simulink model "Reforce_Experiment_FCS"  (R2021a)
settings: Solver=FixedStepDiscrete  StartTime=0.0  StopTime=Inf  FixedStep=Ts  RelTol=1e-3
PostLoadFcn:
  | , if any(exist('dsrtsu_mdlpostloadfcn', 'file') ~= 0), dsrtsu_mdlpostloadfcn('Execute', bdroot); end,
InitFcn:
  | , if any(exist('rtifpga_mdlclblib', 'file') ~= 0), rtifpga_mdlclblib('Init', bdroot); end,
model workspace (MAT data in the model file):
  FPGA_Control_Scheme_1_Buffer_1_1_1_write : Simulink.Signal (value not decoded)
  FPGA_Control_Scheme_1_Buffer_2_1_1_write : Simulink.Signal (value not decoded)
  FPGA_Control_Scheme_1_Register_1_1_1_write : Simulink.Signal (value not decoded)
  FPGA_Control_Scheme_1_Register_2_1_1_write : Simulink.Signal (value not decoded)
values from neighbouring files (symbols this model uses):
  abc2alphabeta0 = [      2/3      -1/3       -1/3 ... (first row only)    [Reforce_Init_FCS.m]
  alphabeta02abc = [  1          0 1/sqrt(2) ... (first row only)    [Reforce_Init_FCS.m]
  torque_ref_sample_lower = -torque_ref_sample_upper    (= -6.5)    [Reforce_Init_FCS.m]
  torque_ref_sample_upper = 6.5    [Reforce_Init_FCS.m]
  Ts = 50e-6    (= 5e-05)    [Reforce_Init_FCS.m]
  uf_factor = U_nom / f_nom    (= 2.82)    [Reforce_Init_FCS.m]
undefined symbols (not defined in the file or in its folder): CC, controller, init_layer_0, init_layer_1, init_layer_2, init_layer_3, init_layer_4, init_layer_5, init_layer_6, init_layer_7, init_layer_8, init_layer_9, inverter, load, motor, PLL, sensor
libraries: simulink x16, rtiproclib x13, rti1202lib_adc_class1 x8, rti1202lib_dio_class1 x4, dspfdesign x3, rtiemclib x2, rti1202lib_dac_class1 x1, embmathops x1, rti1202lib_base x1, rtitasklib x1, dsextras x1, simulink_extras x1
(part 2 of 6)

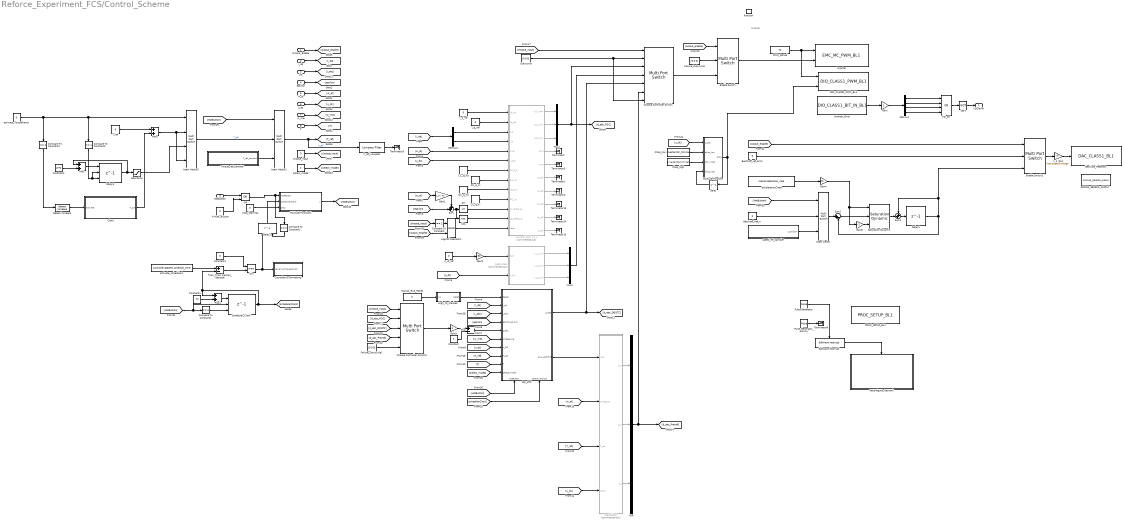
== system Reforce_Experiment_FCS/Control_Scheme ==
  note: Inverter
  Output_Enable : Inport
  i_dq : Inport  Port=2
  In3 : Inport  Port=3
  epsilon : Inport  Port=4
  w_el : Inport  Port=5
  u_dc : Inport  Port=6
  w_me : Inport  Port=7
  T : Inport  Port=8
  HotButton : Inport  Port=9
  function : TriggerPort  TriggerType=function-call  VariantControl=(inherit)
  Add : Sum
  Add1 : Sum
  Beckhoff_Ref_n : Constant  Value=0
  Beckhoff_Referenz : rti1202lib_dac_class1/DAC_CLASS1_BL1  DSProperties=struct('RTI',struct('Version',uint32(2),'BlockType',struct('isSLSource',uint8(0),'isSLSink',uint8(1),'isHWSource',uint8(0),'isHWSink',uint8(1),'isSetup',uint8(0),'isInline',uint8(1),'isNonInline',uint8(0),'isInterrupt',uint8(0),'isChannelwise',uint8(1)),'IOBoardType',{{'DS120X','STD','DACC1'}},'UnitType','DAC','Identifier','DAC','DialogType','ML','BlockSet','NONE','SlaveProcessor','NONE'))  RTIBlockInterface=struct('InputPortsActive',1,'InputPortsWidth',int32(1),'InputPortsDataType',{{'SS_DOUBLE'}},'InputPortsName',{{['DAC 8']}},'DialogFcn','rti120xstddacc1dacgui','InitLevel',3,'IconTransparency','on','BlockDisplay',{{['DAC CL1\nChannel: 8'],'center'}},'BlockName',struct('Token',{{'DAC_CLASS1_BL1'}}))  RTIBlockParameters=struct('ChannelNo',{{8,'OFF',[]}},'ChannelNumOf',{{1,'OFF',[]}},'InitialValue1',{{'0','OFF',[-10 10]}},'InitialValue2',{{'0','OFF',[-10 10]}},'InitialValue3',{{'0','OFF',[-10 10]}},'InitialValue4',{{'0','OFF',[-10 10]}},'InitialValue5',{{'0','OFF',[-10 10]}},'InitialValue6',{{'0','OFF',[-10 10]}},'InitialValue7',{{'0','OFF',[-10 10]}},'InitialValue8',{{'0','OFF',[-10 10]}},'InitialValue9',{{'0','OFF',[-10 10]}},'InitialValue10',{{'0','OFF',[-10 10]}},'InitialValue11',{{'0','OFF',[-10 10]}},'InitialValue12',{{'0','OFF',[-10 10]}},'InitialValue13',{{'0','OFF',[-10 10]}},'InitialValue14',{{'0','OFF',[-10 10]}},'InitialValue15',{{'0','OFF',[-10 10]}},'InitialValue16',{{'0','OFF',[-10 10]}},'OutputMode',{{[2 1 1 1 1 1 1 1 1 1 1 1 1 1 1 1],'OFF',[1 2]}},'TermValue1',{{'0','OFF',[-10 10]}},'TermValue2',{{'0','OFF',[-10 10]}},'TermValue3',{{'0','OFF',[-10 10]}},'TermValue4',{{'0','OFF',[-10 10]}},'TermValue5',{{'0','OFF',[-10 10]}},'TermValue6',{{'0','OFF',[-10 10]}},'TermValue7',{{'0','OFF',[-10 10]}},'TermValue8',{{'0','OFF',[-10 10]}},'TermValue9',{{'0','OFF',[-10 10]}},'TermValue10',{{'0','OFF',[-10 10]}},'TermValue11',{{'0','OFF',[-10 10]}},'TermValue12',{{'0','OFF',[-10 10]}},'TermValue13',{{'0','OFF',[-10 10]}},'TermValue14',{{'0','OFF',[-10 10]}},'TermValue15',{{'0','OFF',[-10 10]}},'TermValue16',{{'0','OFF',[-10 10]}},'EnableTermMode',{{1,'OFF',[0 1]}},'TLCFileName',{{'rti120xdac_c1_dac','OFF',[]}},'InitialValueBuildCheck1',{{0,'OFF',[]}},'InitialValueBuildCheck2',{{0,'OFF',[]}},'InitialValueBuildCheck3',{{0,'OFF',[]}},'InitialValueBuildCheck4',{{0,'OFF',[]}},'InitialValueBuildCheck5',{{0,'OFF',[]}},'InitialValueBuildCheck6',{{0,'OFF',[]}},'InitialValueBuildCheck7',{{0,'OFF',[]}},'InitialValueBuildCheck8',{{1,'OFF',[]}},'InitialValueBuildCheck9',{{0,'OFF',[]}},'InitialValueBuildCheck10',{{0,'OFF',[]}},'InitialValueBuildCheck11',{{0,'OFF',[]}},'InitialValueBuildCheck12',{{0,'OFF',[]}},'InitialValueBuildCheck13',{{0,'OFF',[]}},'InitialValueBuildCheck14',{{0,'OFF',[]}},'InitialValueBuildCheck15',{{0,'OFF',[]}},'InitialValueBuildCheck16',{{0,'OFF',[]}},'TermValueBuildCheck1',{{0,'OFF',[]}},'TermValueBuildCheck2',{{0,'OFF',[]}},'TermValueBuildCheck3',{{0,'OFF',[]}},'TermValueBuildCheck4',{{0,'OFF',[]}},'TermValueBuildCheck5',{{0,'OFF',[]}},'TermValueBuildCheck6',{{0,'OFF',[]}},'TermValueBuildCheck7',{{0,'OFF',[]}},'TermValueBuildCheck8',{{0,'OFF',[]}},'TermValueBuildCheck9',{{0,'OFF',[]}},'TermValueBuildCheck10',{{0,'OFF',[]}},'TermValueBuildCheck11',{{0,'OFF',[]}},'TermValueBuildCheck12',{{0,'OFF',[]}},'TermValueBuildCheck13',{{0,'OFF',[]}},'TermValueBuildCheck14',{{0,'OFF',[]}},'TermValueBuildCheck15',{{0,'OFF',[]}},'TermValueBuildCheck16',{{0,'OFF',[]}})  RTISFcnParameters=struct('ChannelNo','int16','ChannelNumOf','int16','InitialValue1','double','InitialValue2','double','InitialValue3','double','InitialValue4','double','InitialValue5','double','InitialValue6','double','InitialValue7','double','InitialValue8','double','InitialValue9','double','InitialValue10','double','InitialValue11','double','InitialValue12','double','InitialValue13','double','InitialValue14','double','InitialValue15','double','InitialValue16','double','OutputMode','int16','TermValue1','double','TermValue2','double','TermValue3','double','TermValue4','double','TermValue5','double','TermValue6','double','TermValue7','double','TermValue8','double','TermValue9','double','TermValue10','double','TermValue11','double','TermValue12','double','TermValue13','double','TermValue14','double','TermValue15','double','TermValue16','double','EnableTermMode','int16','TLCFileName','char')  RTIBlockParaDefault=struct('ChannelNo',1,'ChannelNumOf',1,'InitialValue1',0,'InitialValue2',0,'InitialValue3',0,'InitialValue4',0,'InitialValue5',0,'InitialValue6',0,'InitialValue7',0,'InitialValue8',0,'InitialValue9',0,'InitialValue10',0,'InitialValue11',0,'InitialValue12',0,'InitialValue13',0,'InitialValue14',0,'InitialValue15',0,'InitialValue16',0,'OutputMode',ones(1,16),'TermValue1',0,'TermValue2',0,'TermValue3',0,'TermValue4',0,'TermValue5',0,'TermValue6',0,'TermValue7',0,'TermValue8',0,'TermValue9',0,'TermValue10',0,'TermValue11',0,'TermValue12',0,'TermValue13',0,'TermValue14',0,'TermValue15',0,'TermValue16',0,'EnableTermMode',0,'TLCFileName','rti120xdac_c1_dac','InitialValueBuildCheck1',0,'InitialValueBuildCheck2',0,'InitialValueBuildCheck3',0,'InitialValueBuildCheck4',0,'InitialValueBuildCheck5',0,'InitialValueBuildCheck6',0,'InitialValueBuildCheck7',0,'InitialValueBuildCheck8',0,'InitialValueBuildCheck9',0,'InitialValueBuildCheck10',0,'InitialValueBuildCheck11',0,'InitialValueBuildCheck12',0,'InitialValueBuildCheck13',0,'InitialValueBuildCheck14',0,'InitialValueBuildCheck15',0,'InitialValueBuildCheck16',0,'TermValueBuildCheck1',0,'TermValueBuildCheck2',0,'TermValueBuildCheck3',0,'TermValueBuildCheck4',0,'TermValueBuildCheck5',0,'TermValueBuildCheck6',0,'TermValueBuildCheck7',0,'TermValueBuildCheck8',0,'TermValueBuildCheck9',0,'TermValueBuildCheck10',0,'TermValueBuildCheck11',0,'TermValueBuildCheck12',0,'TermValueBuildCheck13',0,'TermValueBuildCheck14',0,'TermValueBuildCheck15',0,'TermValueBuildCheck16',0)
  Beckhoff_ref_error : Constant  Value=0
  CC_d_Ki : Constant  Value=CC.d.Ki
  CC_d_Kp : Constant  Value=CC.d.Kp
  CC_q_Ki : Constant  Value=CC.q.Ki
  CC_q_Kp : Constant  Value=CC.q.Kp
  Chart : Stateflow chart  TreatAsAtomicUnit=on
  Choose Controller Switch : MultiPortSwitch  DataPortOrder=Zero-based contiguous  Inputs=5  DataPortForDefault=Additional data port  zeroidx=on
  Choose Controller Switch1 : MultiPortSwitch  DataPortOrder=Specify indices  Inputs=5  DataPortIndices={1,3,4}  DataPortForDefault=Additional data port  DiagnosticForDefault=None
  Chop_high : Constant  Value=inverter.DC_link.high
  Chop_low : Constant  Value=inverter.DC_link.low
  Compare To Constant : simulink/Logic and Bit Operations/Compare To Constant  relop===  const=1  OutDataTypeStr=boolean
  Compare To Constant1 : simulink/Logic and Bit Operations/Compare To Constant  relop===  const=0  OutDataTypeStr=boolean
  Compare To Constant2 : simulink/Logic and Bit Operations/Compare To Constant  relop===  const=0  OutDataTypeStr=boolean
  Compare To Constant3 : simulink/Logic and Bit Operations/Compare To Constant  relop===  const=1  OutDataTypeStr=boolean
  Compare To Constant4 : simulink/Logic and Bit Operations/Compare To Constant  relop===  const=2  OutDataTypeStr=boolean
  Constant : Constant
  Constant1 : Constant  Value=Ts
  Constant2 : Constant  Value=4*Ts
  Constant4 : Constant  Value=0
  Cos : Trigonometry  Operator=cos  NumberOfDataPoints=64
  Countdown_Formatting : Subsystem
  DIO_CLASS1_PWM_BL1 : rti1202lib_dio_class1/DIO_CLASS1_PWM_BL1  DSProperties=struct('RTI',struct('Version',uint32(1),'BlockType',struct('isSLSource',uint8(0),'isSLSink',uint8(1),'isHWSource',uint8(0),'isHWSink',uint8(1),'isSetup',uint8(0),'isInline',uint8(1),'isNonInline',uint8(0),'isInterrupt',uint8(0),'isChannelwise',uint8(1)),'IOBoardType',{{'DS120X','STD','DIOC1'}},'UnitType','PWM','Identifier','PWM','DialogType','ML','BlockSet','NONE','SlaveProcessor','NONE'))  RTIBlockInterface=struct('InputPortsWidth',int32([1 1]),'InputPortsActive',[1 1],'InputPortsName',{{'Period',['Duty Cycle']}},'BlockDisplay',{{['DIO CL1 PWM\nPort: 1\nChannel: 7'],'center'}},'IconTransparency','on','InitLevel',3,'DialogFcn','rti120xstddioc1pwmgui','BlockName',struct('Token',{{'DIO_CLASS1_PWM_BL1'}}))  RTIBlockParameters=struct('PortNo',{{1,'OFF',[]}},'ChannelNo',{{7,'OFF',[]}},'HighLevel',{{2,'OFF',[1 3]}},'UpdateMode',{{1,'OFF',[1 2]}},'InvertingMode',{{1,'OFF',[1 2]}},'DutyCycleInit',{{'0.0','OFF',[0 1]}},'DutyCycleTerm',{{'0','OFF',[0 1]}},'PeriodInit',{{'Ts','OFF',[1e-7 1.34]}},'PeriodTerm',{{'Ts','OFF',[1e-7 1.34]}},'TerminationMode',{{1,'OFF',[0 1]}},'OutputTermValidate',{{1,'OFF',[0 1]}},'OutputTermBuildCheck',{{true,'OFF',[]}},'EnableEvent',{{0,'OFF',[0 1]}},'EventMode',{{1,'OFF',[1 3]}},'EventOnFalling',{{1,'OFF',[0 1]}},'EventOnRising',{{0,'OFF',[0 1]}},'EventDelay',{{'0','OFF',[0 1.34]}},'EventRate',{{'1','OFF',[1 256]}},'EventBuildCheck',{{false,'OFF',[]}},'TriggerLine',{{1,'OFF',[1 16]}},'TLCFileName',{{'rti120xdio_c1_pwm','OFF',[]}})  RTISFcnParameters=struct('PortNo','int16','ChannelNo','int16','HighLevel','int16','UpdateMode','int16','InvertingMode','int16','DutyCycleInit','double','DutyCycleTerm','double','PeriodInit','double','PeriodTerm','double','TerminationMode','int16','OutputTermValidate','int16','EnableEvent','int16','EventMode','int16','EventOnFalling','int16','EventOnRising','int16','EventDelay','double','EventRate','int16','TriggerLine','int16','TLCFileName','char')  RTIBlockParaDefault=struct('PortNo',1,'ChannelNo',1,'HighLevel',1,'UpdateMode',1,'InvertingMode',1,'DutyCycleInit',2^-1,'DutyCycleTerm',2^-1,'PeriodInit',5e-5,'PeriodTerm',5e-5,'TerminationMode',0,'OutputTermValidate',0,'OutputTermBuildCheck',0,'EnableEvent',0,'EventMode',1,'EventOnFalling',1,'EventOnRising',0,'EventDelay',0,'EventRate',1,'EventBuildCheck',0,'TriggerLine',1,'TLCFileName','rti120xdio_c1_pwm')
  DQ_DTC : Subsystem
      settings: PortSchema="{\"entries\":[{\"content\":{\"sides\":[{\"content\":{\"connectorIds\":[\"In1\",\"In2\",\"In3\",\"In4\",\"In5\",\"In6\",\"In7\",\"In8\",\"In9\",\"In10\"]},\"type\":\"ConnectorPlacement.EquallySpacedRectSide\",\"uuid\":\"02ff152a-d5e9-48ae-8ae9-04f46c283eee\"},{\"content\":{\"connectorIds\":[\"Out1\",\"Out2\"],\"side\":\"RIGHT\"},\"type\":\"ConnectorPlacement.EquallySpacedRectSide\",\"uuid\":\"642da27a-b041-4256-941e-23b0305d4ed5\"},{\"content\":{\"connectorIds\":[],\"side\":\"TOP\"},\"type\":\"ConnectorPlacement.EquallySpacedRectSide\",\"uuid\":\"a1b72579-caca-49f6-8122-3333a1b1b672\"},{\"content\":{\"connectorIds\":[\"In11\",\"In12\"],\"side\":\"BOTTOM\"},\"type\":\"ConnectorPlacement.EquallySpacedRectSide\",\"uuid\":\"d4b983f3-21ae-48af-86f0-0aec95f79f6c\"}]},\"type\":\"ConnectorPlacement.EquallySpacedConnector\",\"uuid\":\"9d77db4d-e82d-471c-b407-1ac7a7d31965\"}],\"packageUris\":[\"http://schema.mathworks.com/mf0/Connector/R2020b\"],\"version\":\"1.0\"}"
  DS1202_SENSOR_SUPPLY : rti1202lib_base/DS1202_SENSOR_SUPPLY  DSProperties=struct('RTI',struct('Version',uint32(1),'BlockType',struct('isSLSource',uint8(0),'isSLSink',uint8(0),'isHWSource',uint8(0),'isHWSink',uint8(1),'isSetup',uint8(0),'isInline',uint8(1),'isNonInline',uint8(0),'isInterrupt',uint8(0),'isChannelwise',uint8(0)),'IOBoardType',{{'DS120X','BASE'}},'UnitType','SENSORSUPPLY','Identifier','SENSORSUPPLY','DialogType','ML','BlockSet','NONE','SlaveProcessor','NONE'))  RTIBlockInterface=struct('OutputPortsActive',0,'OutputPortsWidth',int32(0),'DialogFcn','rti120xbasesensorsupplygui','InitLevel',3,'IconTransparency','off','BlockDisplay',{{['DS1202\nSensor Supply'],'center'}},'BlockName',struct('Token',{{'DS1202_SENSOR_SUPPLY'}}))  RTIBlockParameters=struct('Voltage',{{2,'OFF',[2 20]}},'TLCFileName',{{'rti120xbase_sensor_supply','OFF',[]}})  RTISFcnParameters=struct('Voltage','double','TLCFileName','char')  RTIBlockParaDefault=struct('Voltage',2,'TLCFileName','rti120xbase_sensor_supply')
  Delay : Delay  DelayLength=1
  Delay1 : Delay  DelayLength=1  InitialCondition=0
  Delay2 : Delay  DelayLength=1  InitialCondition=controller.DQDTC.schedule_time  ExternalReset=Either
      settings: InputPortMap=u0,r5
  Delay3 : Delay  DelayLength=1  InitialCondition=-5  ExternalReset=Either  ShowEnablePort=on
      settings: InputPortMap=u0,e6,r5
  Demux1 : Demux
  Demux2 : Demux  Outputs=2
  Detect Increase : simulink/Logic and Bit Operations/Detect Increase  vinit=0.0  OutDataTypeStr=boolean
  Dutycycle : Constant  Value=[0 0 0]
  Enable Switch : MultiPortSwitch  DataPortOrder=Zero-based contiguous  Inputs=2  zeroidx=on
  Enable Switch1 : MultiPortSwitch  DataPortOrder=Zero-based contiguous  Inputs=2  zeroidx=on
  Failure_Dutycycle : Constant  Value=[0 0 0]
  Failure_Dutycycle1 : Constant  Value=[0 0 0]
  Gain : Gain
  Gain1 : Gain  Gain=1.5 * Ts
  Gain2 : Gain  Gain=60
  Gain3 : Gain  Gain=2
  Gain4 : Gain  Gain=Ts
  Gain5 : Gain  Gain=-1
  High_To_Flanke3 : Subsystem
  Index Vector : MultiPortSwitch  DataPortOrder=Zero-based contiguous  Inputs=2  zeroidx=on
  Index Vector1 : MultiPortSwitch  DataPortOrder=Zero-based contiguous  Inputs=2  zeroidx=on
  Index Vector2 : MultiPortSwitch  DataPortOrder=Zero-based contiguous  zeroidx=on
  Inverter : rtiemclib/EMC_MC_PWM_BL1  DSProperties=struct('RTI',struct('Version',uint32(2),'BlockType',struct('isSLSource',uint8(0),'isSLSink',uint8(1),'isHWSource',uint8(0),'isHWSink',uint8(1),'isSetup',uint8(0),'isInline',uint8(1),'isNonInline',uint8(0),'isInterrupt',uint8(0),'isChannelwise',uint8(1)),'IOBoardType','DSEMC','UnitType','MCPWM','Identifier','MCPWM','DialogType','ML','BlockSet','RTIEMC','SlaveProcessor','NONE'))  RTIBlockInterface=struct('InputPortsWidth',int32([1 3 1]),'InputPortsActive',[1 1 0],'InputPortsName',{{'Period',['Duty Cycle'],['Output Enable']}},'BlockDisplay',{{['EMC Multi Channel PWM\nPort: 1\nChannel: 1\nNumber of channels: 3'],'center'}},'IconTransparency','on','InitLevel',3,'DialogFcn','rtiemcmcpwmgui','BlockName',struct('Token',{{'EMC_MC_PWM_BL1'}}),'InputPortsDataType',{{'SS_DOUBLE','SS_DOUBLE','SS_BOOLEAN'}})  RTIBlockParameters=struct('PortNo',{{1,'OFF',[1 3]}},'ChannelNo',{{1,'OFF',[1 16]}},'InvChannelMode',{{2,'OFF',[1 2]}},'NumOfChannels',{{3,'OFF',[1 8]}},'HighLevel',{{2,'OFF',[1 3]}},'AlignmentMode',{{2,'OFF',[1 2]}},'UpdateModeCA',{{1,'OFF',[1 3]}},'UpdateModeEA',{{2,'OFF',[1 2]}},'DeadTime',{{'5e-6','OFF',[0 0.000655]}},'InitPeriod',{{'50e-6','OFF',[1e-7 1.34]}},'InitDutyCycle1',{{'0','OFF',[0 1]}},'InitDutyCycle2',{{'0','OFF',[0 1]}},'InitDutyCycle3',{{'0','OFF',[0 1]}},'InitDutyCycle4',{{'0.5','OFF',[0 1]}},'InitDutyCycle5',{{'0.5','OFF',[0 1]}},'InitDutyCycle6',{{'0.5','OFF',[0 1]}},'InitDutyCycle7',{{'0.5','OFF',[0 1]}},'InitDutyCycle8',{{'0.5','OFF',[0 1]}},'InitDutyCycle9',{{'0.5','OFF',[0 1]}},'InitDutyCycle10',{{'0.5','OFF',[0 1]}},'InitDutyCycle11',{{'0.5','OFF',[0 1]}},'InitDutyCycle12',{{'0.5','OFF',[0 1]}},'InitDutyCycle13',{{'0.5','OFF',[0 1]}},'InitDutyCycle14',{{'0.5','OFF',[0 1]}},'InitDutyCycle15',{{'0.5','OFF',[0 1]}},'InitDutyCycle16',{{'0.5','OFF',[0 1]}},'TerminationMode',{{1,'OFF',[0 1]}},'OutputTermValidate',{{1,'OFF',[0 1]}},'TermPeriod',{{'50e-06','OFF',[1e-7 1.34]}},'TermDutyCycle1',{{'0','OFF',[0 1]}},'TermDutyCycle2',{{'0','OFF',[0 1]}},'TermDutyCycle3',{{'0','OFF',[0 1]}},'TermDutyCycle4',{{'0.5','OFF',[0 1]}},'TermDutyCycle5',{{'0.5','OFF',[0 1]}},'TermDutyCycle6',{{'0.5','OFF',[0 1]}},'TermDutyCycle7',{{'0.5','OFF',[0 1]}},'TermDutyCycle8',{{'0.5','OFF',[0 1]}},'TermDutyCycle9',{{'0.5','OFF',[0 1]}},'TermDutyCycle10',{{'0.5','OFF',[0 1]}},'TermDutyCycle11',{{'0.5','OFF',[0 1]}},'TermDutyCycle12',{{'0.5','OFF',[0 1]}},'TermDutyCycle13',{{'0.5','OFF',[0 1]}},'TermDutyCycle14',{{'0.5','OFF',[0 1]}},'TermDutyCycle15',{{'0.5','OFF',[0 1]}},'TermDutyCycle16',{{'0.5','OFF',[0 1]}},'EnableEvent',{{0,'OFF',[0 1]}},'EventMode',{{3,'OFF',[1 3]}},'EventOnStart',{{1,'OFF',[0 1]}},'EventOnCenter',{{0,'OFF',[0 1]}},'EventDelay',{{'25e-6','OFF',[0 1.34]}},'EventRate',{{'1','OFF',[1 256]}},'TriggerLine',{{1,'OFF',[1 16]}},'TLCFileName',{{'rtiemcmcpwm','OFF',[]}},'ValidateDeadTimeBuildCheck',{{false,'OFF',[]}},'InitDutyCycleBuildCheck1',{{1,'OFF',[]}},'InitDutyCycleBuildCheck2',{{1,'OFF',[]}},'InitDutyCycleBuildCheck3',{{1,'OFF',[]}},'InitDutyCycleBuildCheck4',{{0,'OFF',[]}},'InitDutyCycleBuildCheck5',{{0,'OFF',[]}},'InitDutyCycleBuildCheck6',{{0,'OFF',[]}},'InitDutyCycleBuildCheck7',{{0,'OFF',[]}},'InitDutyCycleBuildCheck8',{{0,'OFF',[]}},'InitDutyCycleBuildCheck9',{{0,'OFF',[]}},'InitDutyCycleBuildCheck10',{{0,'OFF',[]}},'InitDutyCycleBuildCheck11',{{0,'OFF',[]}},'InitDutyCycleBuildCheck12',{{0,'OFF',[]}},'InitDutyCycleBuildCheck13',{{0,'OFF',[]}},'InitDutyCycleBuildCheck14',{{0,'OFF',[]}},'InitDutyCycleBuildCheck15',{{0,'OFF',[]}},'InitDutyCycleBuildCheck16',{{0,'OFF',[]}},'ValidateTermBuildCheck',{{true,'OFF',[]}},'TermDutyCycleBuildCheck1',{{1,'OFF',[]}},'TermDutyCycleBuildCheck2',{{1,'OFF',[]}},'TermDutyCycleBuildCheck3',{{1,'OFF',[]}},'TermDutyCycleBuildCheck4',{{0,'OFF',[]}},'TermDutyCycleBuildCheck5',{{0,'OFF',[]}},'TermDutyCycleBuildCheck6',{{0,'OFF',[]}},'TermDutyCycleBuildCheck7',{{0,'OFF',[]}},'TermDutyCycleBuildCheck8',{{0,'OFF',[]}},'TermDutyCycleBuildCheck9',{{0,'OFF',[]}},'TermDutyCycleBuildCheck10',{{0,'OFF',[]}},'TermDutyCycleBuildCheck11',{{0,'OFF',[]}},'TermDutyCycleBuildCheck12',{{0,'OFF',[]}},'TermDutyCycleBuildCheck13',{{0,'OFF',[]}},'TermDutyCycleBuildCheck14',{{0,'OFF',[]}},'TermDutyCycleBuildCheck15',{{0,'OFF',[]}},'TermDutyCycleBuildCheck16',{{0,'OFF',[]}},'ValidateEventBuildCheck',{{false,'OFF',[]}},'ActivateOutputEnablePort',{{0,'OFF',[0 1]}},'InitOutputEnable',{{2,'OFF',[1 2]}})  RTISFcnParameters=struct('PortNo','int32','ChannelNo','int32','InvChannelMode','int32','NumOfChannels','int32','HighLevel','int32','AlignmentMode','int32','UpdateModeCA','int32','UpdateModeEA','int32','DeadTime','double','InitPeriod','double','InitDutyCycle1','double','InitDutyCycle2','double','InitDutyCycle3','double','InitDutyCycle4','double','InitDutyCycle5','double','InitDutyCycle6','double','InitDutyCycle7','double','InitDutyCycle8','double','InitDutyCycle9','double','InitDutyCycle10','double','InitDutyCycle11','double','InitDutyCycle12','double','InitDutyCycle13','double','InitDutyCycle14','double','InitDutyCycle15','double','InitDutyCycle16','double','TerminationMode','uint32','OutputTermValidate','int32','TermPeriod','double','TermDutyCycle1','double','TermDutyCycle2','double','TermDutyCycle3','double','TermDutyCycle4','double','TermDutyCycle5','double','TermDutyCycle6','double','TermDutyCycle7','double','TermDutyCycle8','double','TermDutyCycle9','double','TermDutyCycle10','double','TermDutyCycle11','double','TermDutyCycle12','double','TermDutyCycle13','double','TermDutyCycle14','double','TermDutyCycle15','double','TermDutyCycle16','double','EnableEvent','int32','EventMode','int32','EventOnStart','int32','EventOnCenter','int32','EventDelay','double','EventRate','int32','TriggerLine','int32','TLCFileName','char','ActivateOutputEnablePort','int32','InitOutputEnable','int32')  RTIBlockParaDefault=struct('PortNo',1,'ChannelNo',1,'InvChannelMode',1,'NumOfChannels',1,'HighLevel',1,'AlignmentMode',1,'UpdateModeCA',1,'UpdateModeEA',1,'DeadTime',0,'InitPeriod',5e-5,'InitDutyCycle1',2^-1,'InitDutyCycle2',2^-1,'InitDutyCycle3',2^-1,'InitDutyCycle4',2^-1,'InitDutyCycle5',2^-1,'InitDutyCycle6',2^-1,'InitDutyCycle7',2^-1,'InitDutyCycle8',2^-1,'InitDutyCycle9',2^-1,'InitDutyCycle10',2^-1,'InitDutyCycle11',2^-1,'InitDutyCycle12',2^-1,'InitDutyCycle13',2^-1,'InitDutyCycle14',2^-1,'InitDutyCycle15',2^-1,'InitDutyCycle16',2^-1,'TerminationMode',0,'OutputTermValidate',0,'TermPeriod',5e-5,'TermDutyCycle1',2^-1,'TermDutyCycle2',2^-1,'TermDutyCycle3',2^-1,'TermDutyCycle4',2^-1,'TermDutyCycle5',2^-1,'TermDutyCycle6',2^-1,'TermDutyCycle7',2^-1,'TermDutyCycle8',2^-1,'TermDutyCycle9',2^-1,'TermDutyCycle10',2^-1,'TermDutyCycle11',2^-1,'TermDutyCycle12',2^-1,'TermDutyCycle13',2^-1,'TermDutyCycle14',2^-1,'TermDutyCycle15',2^-1,'TermDutyCycle16',2^-1,'EnableEvent',0,'EventMode',1,'EventOnStart',1,'EventOnCenter',0,'EventDelay',0,'EventRate',1,'TriggerLine',1,'TLCFileName','rtiemcmcpwm','ValidateDeadTimeBuildCheck',0,'InitDutyCycleBuildCheck1',0,'InitDutyCycleBuildCheck2',0,'InitDutyCycleBuildCheck3',0,'InitDutyCycleBuildCheck4',0,'InitDutyCycleBuildCheck5',0,'InitDutyCycleBuildCheck6',0,'InitDutyCycleBuildCheck7',0,'InitDutyCycleBuildCheck8',0,'InitDutyCycleBuildCheck9',0,'InitDutyCycleBuildCheck10',0,'InitDutyCycleBuildCheck11',0,'InitDutyCycleBuildCheck12',0,'InitDutyCycleBuildCheck13',0,'InitDutyCycleBuildCheck14',0,'InitDutyCycleBuildCheck15',0,'InitDutyCycleBuildCheck16',0,'ValidateTermBuildCheck',0,'TermDutyCycleBuildCheck1',0,'TermDutyCycleBuildCheck2',0,'TermDutyCycleBuildCheck3',0,'TermDutyCycleBuildCheck4',0,'TermDutyCycleBuildCheck5',0,'TermDutyCycleBuildCheck6',0,'TermDutyCycleBuildCheck7',0,'TermDutyCycleBuildCheck8',0,'TermDutyCycleBuildCheck9',0,'TermDutyCycleBuildCheck10',0,'TermDutyCycleBuildCheck11',0,'TermDutyCycleBuildCheck12',0,'TermDutyCycleBuildCheck13',0,'TermDutyCycleBuildCheck14',0,'TermDutyCycleBuildCheck15',0,'TermDutyCycleBuildCheck16',0,'ValidateEventBuildCheck',0,'ActivateOutputEnablePort',0,'InitOutputEnable',1)
      settings: SourceProductName=dSPACE RTI Electric Motor Control Blockset
  Inverter_Error : rti1202lib_dio_class1/DIO_CLASS1_BIT_IN_BL1  DSProperties=struct('RTI',struct('Version',uint32(1),'BlockType',struct('isSLSource',uint8(1),'isSLSink',uint8(0),'isHWSource',uint8(1),'isHWSink',uint8(0),'isSetup',uint8(0),'isInline',uint8(1),'isNonInline',uint8(0),'isInterrupt',uint8(0),'isChannelwise',uint8(1)),'IOBoardType',{{'DS120X','STD','DIOC1'}},'UnitType','BIT','Identifier','BITIN','DialogType','ML','BlockSet','NONE','SlaveProcessor','NONE'))  RTIBlockInterface=struct('OutputPortsWidth',int32(4),'OutputPortsDataType',{{'SS_BOOLEAN'}},'OutputPortsActive',1,'OutputPortsName',{{'Out'}},'BlockDisplay',{{['DIO CL1 BIT IN\nPort: 1\nChannel: 8\nNumber of channels: 4'],'center'}},'IconTransparency','on','InitLevel',3,'DialogFcn','rti120xstddioc1bitingui','BlockName',struct('Token',{{'DIO_CLASS1_BIT_IN_BL1'}}))  RTIBlockParameters=struct('PortNo',{{1,'OFF',[]}},'ChannelNo',{{8,'OFF',[]}},'ChannelNumOf',{{4,'OFF',[]}},'EnableNoiseFilter',{{0,'OFF',[0 1]}},'FilterInterval',{{'0','OFF',[0 0.01]}},'FilterIntervalCheck',{{false,'OFF',[]}},'EnableEvent',{{0,'OFF',[0 1]}},'EventMode',{{1,'OFF',[1 3]}},'EventOnFalling',{{1,'OFF',[0 1]}},'EventOnRising',{{0,'OFF',[0 1]}},'EventDelay',{{'0','OFF',[0 1.34]}},'EventRate',{{'1','OFF',[1 256]}},'EventBuildCheck',{{false,'OFF',[]}},'TriggerLine',{{1,'OFF',[1 16]}},'EventChannelNoIdx',{{1,'OFF',[1 16]}},'TLCFileName',{{'rti120xdio_c1_bit_in','OFF',[]}})  RTISFcnParameters=struct('PortNo','int16','ChannelNo','int16','ChannelNumOf','int16','EnableNoiseFilter','int16','FilterInterval','double','EnableEvent','int16','EventMode','int16','EventOnFalling','int16','EventOnRising','int16','EventDelay','double','EventRate','int16','TriggerLine','int16','EventChannelNoIdx','int16','TLCFileName','char')  RTIBlockParaDefault=struct('PortNo',1,'ChannelNo',1,'ChannelNumOf',1,'EnableNoiseFilter',0,'FilterInterval',0,'FilterIntervalCheck',0,'EnableEvent',0,'EventMode',1,'EventOnFalling',1,'EventOnRising',0,'EventDelay',0,'EventRate',1,'EventBuildCheck',0,'TriggerLine',1,'EventChannelNoIdx',1,'TLCFileName','rti120xdio_c1_bit_in')
  Logical Operator1 : Logic  Operator=NAND  AllPortsSameDT=off  OutDataTypeStr=boolean
  MATLAB Function : MATLAB Function  TreatAsAtomicUnit=on
  MATLAB Function1 : MATLAB Function  TreatAsAtomicUnit=on
  Manual_RLS_Reset : Constant  Value=0
  Min : MinMax  Function=max  Inputs=2
  Mux : Mux  Inputs=3
  Mux1 : Mux  Inputs=3
  Mux2 : Mux  Inputs=3
  NOT : Logic  Operator=NOT  IconShape=distinctive  AllPortsSameDT=off  OutDataTypeStr=boolean
  OR : Logic  Operator=OR  IconShape=distinctive  AllPortsSameDT=off  OutDataTypeStr=boolean
  PROC_SETUP_BL1 : rtiproclib/PROC_SETUP_BL1  DSProperties=struct('RTI',struct('Version',uint32(3),'BlockType',struct('isSLSource',uint8(0),'isSLSink',uint8(0),'isHWSource',uint8(0),'isHWSink',uint8(0),'isSetup',uint8(1),'isInline',uint8(1),'isNonInline',uint8(0),'isInterrupt',uint8(0),'isChannelwise',uint8(0)),'IOBoardType','DSPROC','UnitType','SETUP','Identifier','SETUP','DialogType','ML','BlockSet','NONE','SlaveProcessor',''))  RTIBlockInterface=struct('OutputPortsWidth',int32(0),'OutputPortsActive',0,'InitLevel',3,'DialogFcn','rtiprocsetupgui','BlockDisplay',{{['Processor Setup'],'auto'}},'IconTransparency','off','BlockName',struct('Token',{{'PROC_SETUP_BL1'}}))  RTIBlockParameters=struct('NumBoardsUsed',{{1,'OFF',[1 16]}},'ModelMode',{{2,'OFF',[]}},'IniFileList',{{struct('Fullname',{{'C:\Users\Public\RL_Reforce_CCSandFCS\FPGA_Builds\FPGA_FlexIO_10x90_15Inputs.ini'},{'C:\Users\Public\RL_Reforce_CCSandFCS\FPGA_Builds\FPGA_FlexIO_10x90_19Inputs.ini'}},'Filename',{'FPGA_FlexIO_10x90_15Inputs','FPGA_FlexIO_10x90_19Inputs'},'Relname',{{'FPGA_BUILDS\FPGA_FLEXIO_10X90_15INPUTS.INI'},{'FPGA_BUILDS\FPGA_FLEXIO_10X90_19INPUTS.INI'}},'Assigned',{1,0}),'OFF',[]}},'SubsysList',{{struct('SubsysName','','SubsysPath','','SubsysHandle','','SetupBlockHandle','','SetupBlockName','','Filename','','Relname','','IniFilePath','','IniFileName','','IniFileDate','','Assigned',''),'OFF',[]}},'AssignList',{{struct('BoardNumber',{1,2,3,4,5,6,7,8,9,10,11,12,13,14,15,16},'ModelType',{2,0,0,0,0,0,0,0,0,0,0,0,0,0,0,0},'ModelNo',{1,0,0,0,0,0,0,0,0,0,0,0,0,0,0,0},'ProgOption',{1,0,0,0,0,0,0,0,0,0,0,0,0,0,0,0},'IncludeBuild',{0,0,0,0,0,0,0,0,0,0,0,0,0,0,0,0},'IncludeProcAppl',{true,0,0,0,0,0,0,0,0,0,0,0,0,0,0,0}),'OFF',[]}},'ProcSetupHandles',{{-1,'OFF',[]}},'MaxNumBoards',{{16,'OFF',[]}},'ModelPath',{{'C:\Users\Public\RL_Reforce_CCSandFCS','OFF',[]}},'FrameDir',{{[' '],'OFF',[]}},'TLCFileName',{{'rtiprocsetup','OFF',[]}},'IsNewBlock',{{0,'OFF',[]}},'NeedsCodeGen',{{0,'OFF',[]}})  RTISFcnParameters=struct('FrameDir','char','TLCFileName','char')  RTIBlockParaDefault=struct('NumBoardsUsed',1,'ModelMode',1,'IniFileList',struct('Fullname','','Filename','','Relname','','Assigned',''),'SubsysList',struct('SubsysName','','SubsysPath','','SubsysHandle','','SetupBlockHandle','','SetupBlockName','','Filename','','Relname','','IniFilePath','','IniFileName','','IniFileDate','','Assigned',''),'AssignList',struct('BoardNumber','','ModelType','','ModelNo','','ProgOption','','IncludeBuild','','IncludeProcAppl',''),'ProcSetupHandles',-1,'MaxNumBoards',16,'ModelPath',[' '],'FrameDir',[' '],'TLCFileName','rtiprocsetup','IsNewBlock',1,'NeedsCodeGen',0)
      settings: AttributesFormatString=Processor-Build
  PWM_Period : Constant  Value=Ts
  Plus : Sum  Inputs=+-
  Plus1 : Sum
  PreindlMPC : Subsystem  Commented=on
  Pulse Generator : DiscretePulseGenerator  Period=7  SampleTime=-1
  Pulse Generator_dummy : DiscretePulseGenerator  Period=500  SampleTime=-1
  Reconfigure_Network : Subsystem
  Saturation : Saturate  UpperLimit=5  LowerLimit=-5
  Saturation Dynamic : simulink/Discontinuities/Saturation Dynamic  OutMin=[]  OutMax=[]  OutDataTypeStr=Inherit: Same as second input  OutDataType=fixdt(1, 16)  OutScaling=2^-10  DoSatur=off
  Scheduler_Clock : Delay  DelayLength=1  ExternalReset=Either  ShowEnablePort=on
      settings: InputPortMap=u0,e6,r5
  Sin : Trigonometry  NumberOfDataPoints=64
  Software Interrupt : rtitasklib/Software Interrupt  TriggerPort=rising  EnablePort=none  ThBlk=struct('blkh',['Reforce_Experiment_FCS/Control_Scheme/Software Interrupt'],'srcId','SWI1','srcSgnId','SWI1','intervalTmrBlockId',[],'srcSgnName',['Software Trigger'],'srcCpuId','','isSrcCpu',1,'isTargetCpu',1,'srcOnMasterCpu',1,'boardType','','boardTypeNo','','boardNo',1,'intNo',0,'subIntNo',-1,'period',0,'entryPoint','rti_SWI1','blockName',['Software Interrupt'],'taskNameDisplayExt','','taskType','SWINT','groupId','SWINT','hookFcn','NULL','isTimerTaskSrc',0,'service','','mpBlkId','','taskPriorityPreConfig','none','taskPriority',-1,'taskSortWeighting',[],'taskSchedulingPolicy','FCFS','taskOvrPreConfig','none','taskOvrStrategy',1,'taskOvrQueueSize',1,'taskVisibility','on','taskGroupId','','taskGroupDisplayOrder',[],'serviceDynamicGen',0,'disableCodeGen',0,'boardBase','0','noBoardBase','')  TLCFileName=rti_swinterrupt  DialogFcn=[]  Reserved2=[]  Reserved3=[]  Reserved4=[]  DSProperties=struct('RTI',struct('Version',uint32(530),'BlockType',struct('isSLSource',uint8(1),'isSLSink',uint8(1),'isHWSource',uint8(0),'isHWSink',uint8(0),'isSetup',uint8(0),'isInline',uint8(1),'isNonInline',uint8(0),'isInterrupt',uint8(1),'isChannelwise',uint8(0)),'IOBoardType','INTLIB','UnitType','SWINT','Identifier','SWINT','DialogType','SL','BlockSet','NONE','SlaveProcessor','NONE','RelationId',struct('TH',struct('BlockId','SWINT'))))  RTIBlockInterface=struct('OutputPortsActive',1,'OutputPortsWidth',int32(1),'FunctionCall',uint32(0),'OutputPortsName',{{[' ']}},'BlockDisplay',{{['Software Interrupt'],'center'}},'IconTransparency','on','InitLevel',3,'BlockName',struct('Token',{{['Software Interrupt']}}),'TriggerPort',{{'rising'}},'EnablePort',{{'none'}},'MaskDescription',['Makes software-generated interrupts available as trigger sources.'],'Options',{{'SS_OPTION_FORCE_NONINLINED_FCNCALL','SS_OPTION_ASYNCHRONOUS'}},'OutputPortsDataType',{{'SS_FCN_CALL'}})  RTIBlockParameters=struct('TriggerPort',{{2,'OFF',[]}},'EnablePort',{{1,'OFF',[]}},'ThBlk',{{['struct(''blkh'',[''Reforce_Experiment_FCS/Control_Scheme/Software Interrupt''],''srcId'',''SWI1'',''srcSgnId'',''SWI1'',''intervalTmrBlockId'',[],''srcSgnName'',[''Software Trigger''],''srcCpuId'','''',''isSrcCpu'',1,''isTargetCpu'',1,''srcOnMasterCpu'',1,''boardType'','''',''boardTypeNo'','''',''boardNo'',1,''intNo'',0,''subIntNo'',-1,''period'',0,''entryPoint'',''rti_SWI1'',''blockName'',[''Software Interrupt''],''taskNameDisplayExt'','''',''taskType'',''SWINT'',''groupId'',''SWINT'',''hookFcn'',''NULL'',''isTimerTaskSrc'',0,''service'','''',''mpBlkId'','''',''taskPriorityPreConfig'',''none'',''taskPriority'',-1,''taskSortWeighting'',[],''taskSchedulingPolicy'',''FCFS'',''taskOvrPreConfig'',''none'',''taskOvrStrategy'',1,''taskOvrQueueSize'',1,''taskVisibility'',''on'',''taskGroupId'','''',''taskGroupDisplayOrder'',[],''serviceDynamicGen'',0,''disableCodeGen'',0,''boardBase'',''0'',''noBoardBase'','''')'],'OFF',[]}},'TLCFileName',{{'rti_swinterrupt','OFF',[]}})  RTISFcnParameters=struct('TriggerPort','double','EnablePort','double','ThBlk','struct','TLCFileName','char')  RTIBlockParaDefault=struct('TriggerPort',1,'EnablePort',2,'ThBlk',['struct(''srcSgnId'', '''')'],'TLCFileName','rti_swinterrupt')
  Subsystem : Subsystem  Commented=on
  Sum : Sum  Inputs=++|
  Sum1 : Sum  Inputs=|+-
  Sum2 : Sum  Inputs=++|
  T_ref : Constant  Value=0
  T_ref_Lowpass : dspfdesign/Lowpass Filter  FilterType=IIR  DesignForMinimumOrder=on  FilterOrder=50  PassbandFrequency=controller.DQDTC.LP_filter.passband_edge  StopbandFrequency=controller.DQDTC.LP_filter.stopband_edge  PassbandRipple=0.1  StopbandAttenuation=80  InheritSampleRate=off  SampleRate=1/Ts  SimulateUsing=Interpreted execution  roundingMode=Floor  coeffsDataTypeStr=fixdt(1,16)
  Terminator{,1..3,5..6,13..15} (9 alike) : Terminator
  Torque_ref_sampler : Subsystem
  Train_Time_Remain_Seconds : Sum  Inputs=+-
  VSI_err : Logic  Operator=OR  Inputs=4  AllPortsSameDT=off  OutDataTypeStr=boolean
  Virtual_Buzzer : Constant  Value=0
  acceleration_rate : Constant  Value=load.acceleration_rate
  activate_TorqueRamp : Constant  Value=0
  activate_scheduler1 : Constant  Value=controller.DQDTC.schedule_time
  choose_input : Constant  Value=0  OutDataTypeStr=uint8  SampleTime=-1
  current_FOC_v1_2 : Subsystem  Commented=on
  i_d_ref : Constant  Value=0
  i_q_ref : Constant  Value=0
  n_2_DAC : Gain  Gain=load.speed2voltage
  n_uf_ref : Constant  Value=0
  select_model : Constant
  speed_ref_sampler : Subsystem
  stop_learning : Constant  Value=0
  VSI_error : Outport
  wires:
  PWM_Period/1 -> DIO_CLASS1_PWM_BL1/1, Inverter/1
  MATLAB Function/1(chop) -> DIO_CLASS1_PWM_BL1/2, Delay/1
  Inverter_Error/1 -> Gain/1
  Output_Enable/1 -> [output_enable]
  Dutycycle/1 -> Choose Controller Switch/2, Choose Controller Switch/7
  Failure_Dutycycle/1 -> Enable Switch/2
  Enable Switch/1 -> Inverter/2
  VSI_err/1 -> NOT/1
  Demux1/1 -> VSI_err/1
  Demux1/2 -> VSI_err/2
  Demux1/3 -> VSI_err/3
  Demux1/4 -> VSI_err/4
  Gain/1 -> Demux1/1
  NOT/1 -> VSI_error/1
  current_FOC_v1_2/2(U_2_nom) -> Mux1/2
  current_FOC_v1_2/3(U_3_nom) -> Mux1/3
  current_FOC_v1_2/1(U_1_nom) -> Mux1/1
  Demux2/1 -> current_FOC_v1_2/3(i_d)
  Demux2/2 -> current_FOC_v1_2/4(i_q)
  i_d_ref/1 -> current_FOC_v1_2/1(id_ref)
  i_q_ref/1 -> current_FOC_v1_2/2(iq_ref)
  [i_dq] -> Demux2/1
  [u_dc] -> current_FOC_v1_2/6(u_DC)
  Sin/1 -> current_FOC_v1_2/11(sin_theta_el)
  Cos/1 -> current_FOC_v1_2/12(cos_theta_el)
  CC_d_Kp/1 -> current_FOC_v1_2/7(CC_P_d)
  CC_d_Ki/1 -> current_FOC_v1_2/8(CC_I_d)
  CC_q_Kp/1 -> current_FOC_v1_2/9(CC_P_q)
  CC_q_Ki/1 -> current_FOC_v1_2/10("CC_I_q ")
  Choose Controller Switch/1 -> Enable Switch/3
  Mux1/1 -> Choose Controller Switch/3, [d_abc_FOC]
  n_2_DAC/1 -> Beckhoff_Referenz/1
  Logical Operator1/1 -> current_FOC_v1_2/13(reset)
  [w_el] -> current_FOC_v1_2/5(w_el)
  current_FOC_v1_2/4(e_id) -> Terminator/1
  current_FOC_v1_2/5(e_iq) -> Terminator5/1
  current_FOC_v1_2/7(uq_ref) -> Terminator2/1
  current_FOC_v1_2/6(ud_ref) -> Terminator1/1
  current_FOC_v1_2/9(ub_ref) -> Terminator14/1
  current_FOC_v1_2/10(uc_ref) -> Terminator15/1
  current_FOC_v1_2/8(ua_ref) -> Terminator13/1
  [w_el] -> Gain1/1
  Sum/1 -> Cos/1, Sin/1
  Gain1/1 -> Sum/1
  [epsilon] -> Sum/2
  n_uf_ref/1 -> Gain2/1
  [u_dc] -> Subsystem/2(u_dc)
  Gain2/1 -> Subsystem/1(f_uf)
  Mux2/1 -> Choose Controller Switch/4
  Subsystem/3(u_3_nom) -> Mux2/3
  Subsystem/2(u_2_nom) -> Mux2/2
  Subsystem/1(u_1_nom) -> Mux2/1
  Compare To Constant/1 -> Logical Operator1/1
  [output_enable] -> Enable Switch1/1
  Enable Switch1/1 -> n_2_DAC/1
  Beckhoff_ref_error/1 -> Enable Switch1/2
  [i_dq] -> DQ_DTC/2(i_dq)
  [epsilon] -> DQ_DTC/4(epsilon_el out)
  [u_dc] -> DQ_DTC/7(u_DC)
  [w_me] -> DQ_DTC/6(omega_me)
  DQ_DTC/1(d_abc) -> Choose Controller Switch/5, [d_abc_DQDTC]
  [T_ref] -> PreindlMPC/3(T_ref)
  [w_el] -> PreindlMPC/2(omega_el)
  [u_dc] -> PreindlMPC/4(u_DC)
  [T_ref] -> DQ_DTC/8(T_ref)
  DQ_DTC/2(all_i_dq[k+2]) -> PreindlMPC/1(i_dq)
  i_dq/1 -> [i_dq]
  w_el/1 -> [w_el]
  epsilon/1 -> [epsilon]
  u_dc/1 -> [u_dc]
  T/1 -> [T]
  w_me/1 -> [w_me]
  [choose_input] -> Choose Controller Switch/1
  [choose_input] -> Compare To Constant/1
  [output_enable] -> Logical Operator1/2
  choose_input/1 -> [choose_input]
  [output_enable] -> Enable Switch/1
  [choose_input] -> Choose Controller Switch1/1
  [T] -> DQ_DTC/9(T)
  select_model/1 -> [select_model]
  [select_model] -> DQ_DTC/10(select_model)
  Manual_RLS_Reset/1 -> High_To_Flanke3/1(In1)
  High_To_Flanke3/1(Reset) -> DQ_DTC/1(Reset)
  Failure_Dutycycle1/1 -> Choose Controller Switch1/5
  [d_abc_DQDTC] -> Choose Controller Switch1/3
  [d_abc_FOC] -> Choose Controller Switch1/2
  Chop_low/1 -> MATLAB Function/2(chop_low)
  [u_dc] -> MATLAB Function/1(u_DC)
  Delay/1 -> MATLAB Function/4(chop_last)
  Chop_high/1 -> MATLAB Function/3(chop_high)
  In3/1 -> [i_abc]
  [i_abc] -> DQ_DTC/3(i_abc)
  Choose Controller Switch1/1 -> Gain3/1
  Gain3/1 -> Plus/1
  Plus/1 -> DQ_DTC/5(s_abc)
  Constant/1 -> Plus/2
  [d_abc_Preindl] -> Choose Controller Switch1/4
  PreindlMPC/1(d_a) -> Mux/1
  PreindlMPC/2(d_b) -> Mux/2
  PreindlMPC/3(d_c) -> Mux/3
  Mux/1 -> [d_abc_Preindl], Choose Controller Switch/6
  Gain4/1 -> Gain5/1, Saturation Dynamic/1
  Sum1/1 -> Saturation Dynamic/2
  Saturation Dynamic/1 -> Sum2/2
  Index Vector/1 -> Sum1/1
  Sum2/1 -> Delay1/1
  Delay1/1 -> Sum1/2, Enable Switch1/3, Sum2/1
  acceleration_rate/1 -> Gain4/1
  Gain5/1 -> Saturation Dynamic/3
  speed_ref_sampler/1(n_random) -> Index Vector/3
  Beckhoff_Ref_n/1 -> Index Vector/2
  Index Vector1/1 -> T_ref_Lowpass/1, [T_ref]  "T_ref"
  Torque_ref_sampler/1(T_ref_random) -> Index Vector1/3
  [HotButton] -> Index Vector1/1
  T_ref_Lowpass/1 -> Terminator3/1
  [HotButton] -> DQ_DTC/11(HotButton)
  Plus1/1 -> Scheduler_Clock/1
  Scheduler_Clock/1 -> [schedulerClock], Train_Time_Remain_Seconds/2, Plus1/1
  activate_scheduler1/1 -> Train_Time_Remain_Seconds/1
  [HotButton] -> Scheduler_Clock/2, Compare To Constant1/1
  Constant1/1 -> Plus1/2
  Compare To Constant1/1 -> Scheduler_Clock/3
  MATLAB Function1/1(y) -> [HotButton]
  [schedulerClock] -> DQ_DTC/12(schedluerClock)
  Delay2/1 -> MATLAB Function1/2(schedulerClock)
  Train_Time_Remain_Seconds/1 -> Min/2
  Constant4/1 -> Min/1
  Min/1 -> Delay2/1, Countdown_Formatting/1(remain_time_seconds)
  stop_learning/1 -> MATLAB Function1/3(stop)
  Compare To Constant2/1 -> Delay2/2
  OR/1 -> Compare To Constant2/1, MATLAB Function1/1(HotButton)
  Virtual_Buzzer/1 -> OR/2
  HotButton/1 -> OR/1
  Constant2/1 -> Add/2
  Add/1 -> Delay3/1
  Delay3/1 -> Add/1, Saturation/1
  Saturation/1 -> Index Vector2/3
  activate_TorqueRamp/1 -> Compare To Constant4/1, Compare To Constant3/1, Index Vector2/1
  Index Vector2/1 -> Index Vector1/2  "T_ref"
  Software Interrupt/1 -> Reconfigure_Network/Trigger
  Compare To Constant3/1 -> Delay3/2, Delay3/3
  Detect Increase/1 -> Chart/1(activate)
  Compare To Constant4/1 -> Detect Increase/1
  T_ref/1 -> Add1/1
  Add1/1 -> Index Vector2/4, Index Vector2/2
  Chart/1(T_out) -> Add1/2
  Pulse Generator_dummy/1 -> Terminator6/1
  Pulse Generator/1 -> Software Interrupt/Trigger
  [HotButton] -> Index Vector/1

== system Reforce_Experiment_FCS/Error_Detection_and_Memory ==
  err1 : Inport
  err2 : Inport  Port=2
  err3 : Inport  Port=3
  err4 : Inport  Port=4
  err5 : Inport  Port=5
  err6 : Inport  Port=6
  err7 : Inport  Port=7
  err8 : Inport  Port=8
  err9 : Inport  Port=9
  err10 : Inport  Port=10
  Err_Reset : Inport  Port=11
  Logical Operator : Logic  Operator=OR  Inputs=10  AllPortsSameDT=off  OutDataTypeStr=boolean
  Logical Operator1 : Logic  AllPortsSameDT=off  OutDataTypeStr=boolean
  Logical Operator2 : Logic  Operator=NOT  AllPortsSameDT=off  OutDataTypeStr=boolean
  S-R Flip-Flop : simulink_extras/Flip Flops/S-R Flip-Flop  initial_condition=0
  Terminator : Terminator
  PWM_enable : Outport
  wires:
  S-R Flip-Flop/2 -> PWM_enable/1
  Logical Operator1/1 -> S-R Flip-Flop/2
  S-R Flip-Flop/1 -> Terminator/1
  Logical Operator/1 -> S-R Flip-Flop/1, Logical Operator2/1
  err1/1 -> Logical Operator/1
  Err_Reset/1 -> Logical Operator1/2
  Logical Operator2/1 -> Logical Operator1/1
  err2/1 -> Logical Operator/2
  err3/1 -> Logical Operator/3
  err4/1 -> Logical Operator/4
  err5/1 -> Logical Operator/5
  err7/1 -> Logical Operator/7
  err6/1 -> Logical Operator/6
  err8/1 -> Logical Operator/8
  err9/1 -> Logical Operator/9
  err10/1 -> Logical Operator/10
